simulink model "wheelspeed_logic_test"  (R2023b)
settings: Solver=FixedStepAuto  StartTime=0.0  StopTime=20  RelTol=1e-3
settings Model: Creator=Mason Snyder  LastModifiedBy=Mason Snyder

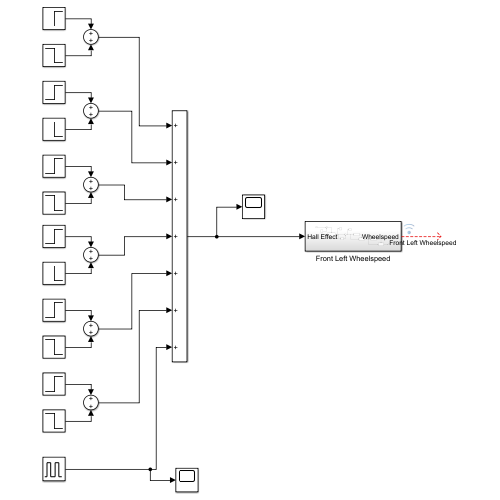
[thumbnail: Simulink's stored preview of the top-level diagram]
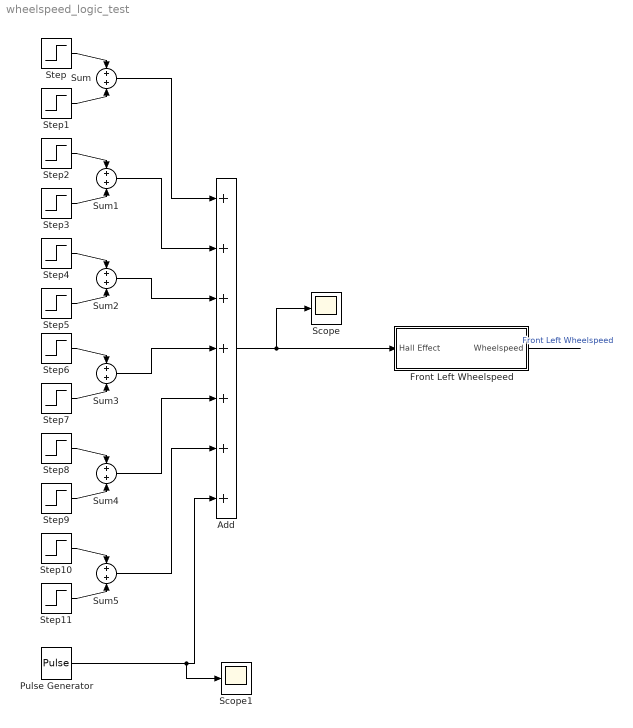
== system wheelspeed_logic_test ==
  Add : Sum  Inputs=+++++++
  Front Left Wheelspeed : Subsystem
  Pulse Generator : DiscretePulseGenerator  PulseType=Time based  Period=1/10  PulseWidth=50  PhaseDelay=7-1/16
  Scope : Scope
  Scope1 : Scope
  Step : Step  SampleTime=0
  Step1 : Step  Time=3  After=-1  SampleTime=0
  Step10 : Step  Time=6.8125  SampleTime=0
  Step11 : Step  Time=6.875  After=-1  SampleTime=0
  Step2 : Step  Time=4  SampleTime=0
  Step3 : Step  Time=5  After=-1  SampleTime=0
  Step4 : Step  Time=5.5  SampleTime=0
  Step5 : Step  Time=6  After=-1  SampleTime=0
  Step6 : Step  Time=6.25  SampleTime=0
  Step7 : Step  Time=6.5  After=-1  SampleTime=0
  Step8 : Step  Time=6.625  SampleTime=0
  Step9 : Step  Time=6.75  After=-1  SampleTime=0
  Sum{,1..5} (6 alike) : Sum  Inputs=+|+
  wires:
  Front Left Wheelspeed/1(Wheelspeed) -> ?  "Front Left Wheelspeed"
  Step/1 -> Sum/1
  Step1/1 -> Sum/2
  Step3/1 -> Sum1/2
  Step2/1 -> Sum1/1
  Step4/1 -> Sum2/1
  Step5/1 -> Sum2/2
  Step7/1 -> Sum3/2
  Step6/1 -> Sum3/1
  Add/1 -> Scope/1, Front Left Wheelspeed/1(Hall Effect)
  Sum2/1 -> Add/3
  Sum3/1 -> Add/4
  Sum1/1 -> Add/2
  Sum/1 -> Add/1
  Step10/1 -> Sum5/1
  Step11/1 -> Sum5/2
  Step9/1 -> Sum4/2
  Step8/1 -> Sum4/1
  Sum4/1 -> Add/5
  Sum5/1 -> Add/6
  Pulse Generator/1 -> Scope1/1, Add/7

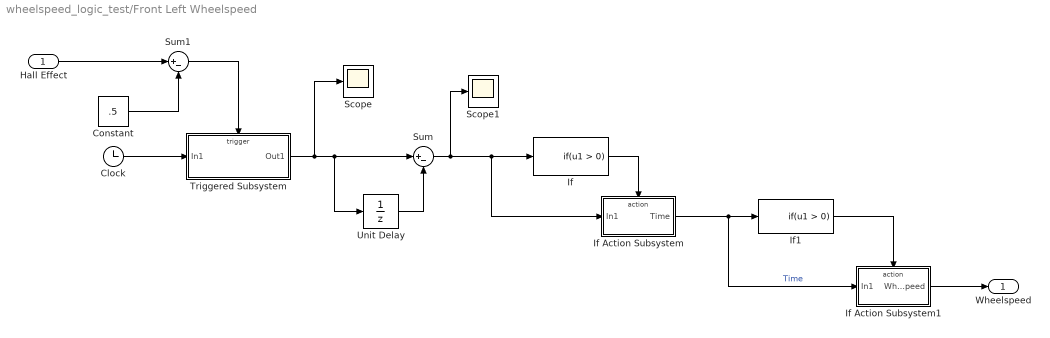
== system wheelspeed_logic_test/Front Left Wheelspeed ==
  Hall Effect : Inport
  Clock : Clock
  Constant : Constant  Value=.5
  If : If  ShowElse=off
  If Action Subsystem : Subsystem  TreatAsAtomicUnit=on
  If Action Subsystem1 : Subsystem  TreatAsAtomicUnit=on
  If1 : If  ShowElse=off
  Scope : Scope
  Scope1 : Scope
  Sum : Sum  Inputs=|+-
  Sum1 : Sum  Inputs=|+-
  Triggered Subsystem : Subsystem  TreatAsAtomicUnit=on
  Unit Delay : UnitDelay  SampleTime=-1  HasFrameUpgradeWarning=on
  Wheelspeed : Outport
  wires:
  Sum1/1 -> Triggered Subsystem/Trigger
  If/1 -> If Action Subsystem/Action
  Sum/1 -> Scope1/1, If Action Subsystem/1(In1), If/1
  Hall Effect/1 -> Sum1/1
  Clock/1 -> Triggered Subsystem/1(In1)
  Unit Delay/1 -> Sum/2
  Triggered Subsystem/1(Out1) -> Scope/1, Sum/1, Unit Delay/1
  Constant/1 -> Sum1/2
  If Action Subsystem/1(Time) -> If Action Subsystem1/1(In1), If1/1  "Time"
  If1/1 -> If Action Subsystem1/Action
  If Action Subsystem1/1(Wheelspeed) -> Wheelspeed/1

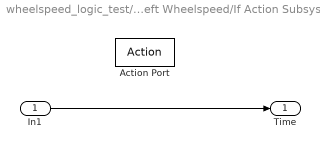
== system wheelspeed_logic_test/Front Left Wheelspeed/If Action Subsystem ==
  In1 : Inport
  Action Port : ActionPort  ActionPortLabel=if(u1 > 0)
  Time : Outport
  wires:
  In1/1 -> Time/1

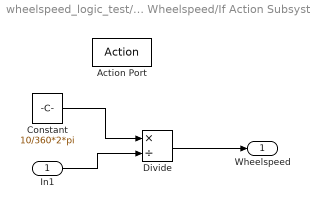
== system wheelspeed_logic_test/Front Left Wheelspeed/If Action Subsystem1 ==
  In1 : Inport
  Action Port : ActionPort  ActionPortLabel=if(u1 > 0)
  Constant : Constant  Value=10/360*2*pi
  Divide : Product  Inputs=*/
  Wheelspeed : Outport
  wires:
  In1/1 -> Divide/2
  Divide/1 -> Wheelspeed/1
  Constant/1 -> Divide/1

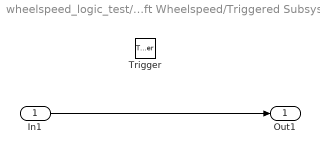
== system wheelspeed_logic_test/Front Left Wheelspeed/Triggered Subsystem ==
  In1 : Inport
  Trigger : TriggerPort  VariantControl=(inherit)
  Out1 : Outport
  wires:
  In1/1 -> Out1/1
